simulink model "cont_desl_scl_16"  (R2016b)
settings: Solver=VariableStepAuto  StartTime=0.0  StopTime=5  RelTol=1e-3
settings Model: Creator=Mateus Gilbert  LastModifiedBy=Mateus Gilbert
settings DataIOCC: ReturnWorkspaceOutputs=on
settings SFSimCC: SimUseLocalCustomCode=on
settings RTWCC: RTWUseLocalCustomCode=on

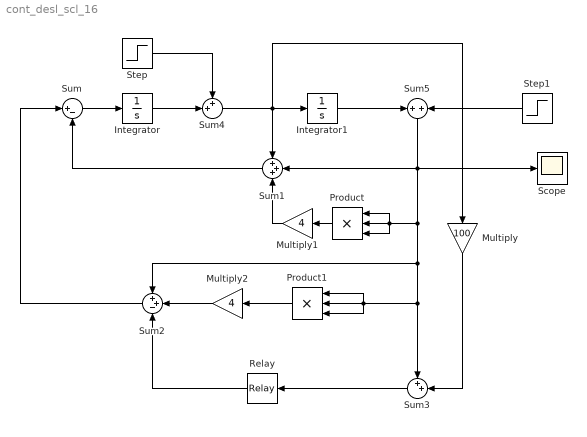
== system cont_desl_scl_16 ==
  Integrator : Integrator
  Integrator1 : Integrator
  Multiply : Gain  Gain=100
  Multiply1 : Gain  Gain=4
  Multiply2 : Gain  Gain=4
  Product : Product  Inputs=3
  Product1 : Product  Inputs=3
  Relay : Relay  OnSwitchValue=1e-5  OffSwitchValue=-1e-5  OffOutputValue=-1
  Scope : Scope
  Step : Step  Time=0  After=9  SampleTime=1e-5
  Step1 : Step  Time=0  After=-2  SampleTime=1e-5
  Sum : Sum  Inputs=|+-
  Sum1 : Sum  Inputs=+++
  Sum2 : Sum  Inputs=++-
  Sum3 : Sum  Inputs=++|
  Sum4 : Sum  Inputs=++|
  Sum5 : Sum  Inputs=+|+
  wires:
  Sum/1 -> Integrator/1
  Sum1/1 -> Sum/2
  Product1/1 -> Multiply2/1
  Relay/1 -> Sum2/3
  Sum3/1 -> Relay/1
  Multiply/1 -> Sum3/2
  Integrator/1 -> Sum4/2
  Sum4/1 -> Integrator1/1, Multiply/1, Sum1/1
  Integrator1/1 -> Sum5/1
  Sum5/1 -> Sum1/2, Product/1, Product/3, Product/2, Sum2/1, Product1/3, Product1/1, Product1/2, Sum3/1, Scope/1
  Product/1 -> Multiply1/1
  Multiply1/1 -> Sum1/3
  Multiply2/1 -> Sum2/2
  Step/1 -> Sum4/1
  Step1/1 -> Sum5/2
  Sum2/1 -> Sum/1
